simulink model "passive_cell_balancing"  (R2017b)
settings: Solver=VariableStepAuto  StartTime=0.0  StopTime=500  MaxStep=1e-4  RelTol=1e-3
undefined symbols (not defined in the file): Hydride, Metal, Nickel
libraries: powerlib x7, electricdrivelib x3
settings Model: Creator=DELL  LastModifiedBy=DELL

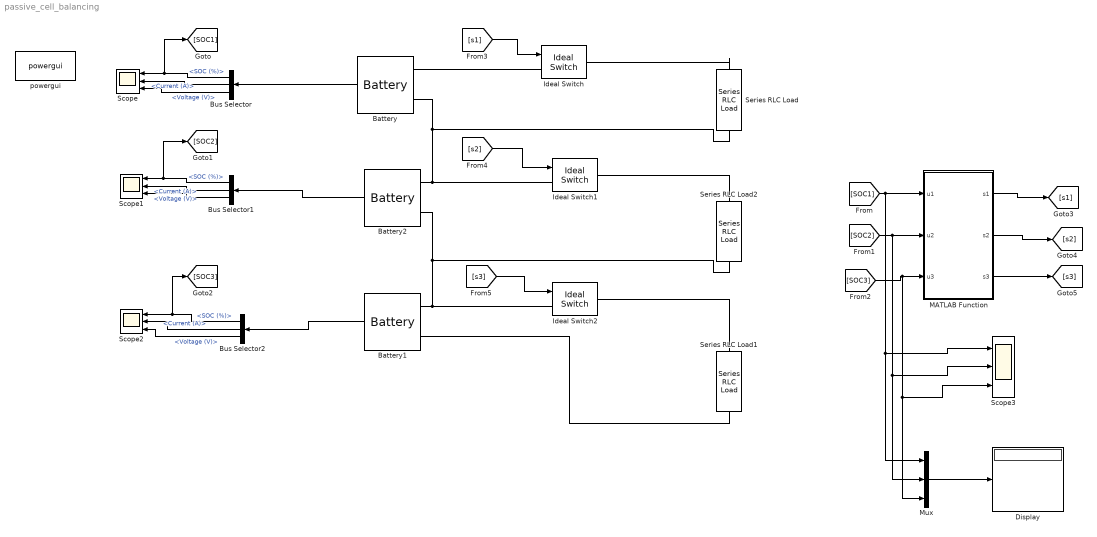
== system passive_cell_balancing ==
  Battery : electricdrivelib/Extra Sources/Battery  BatType=Nickel-Metal-Hydride  ShowTempParam=off  ThermalPreset=no  ShowAgeParam=off  NomV=7.2  NomQ=6.5  SOC=60  Batt_Tr=1  PresetModel=off  MaxQ=5.4  MinV=5.4  FullV=8.3807  Dis_rate=2.3478  R=0.013333  Normal_OP=4.8835  expZone="[7.7788      0.2653]"  current=[6.5 13 32.5]  Units=Time  Tci=20  NomT=20  T2=-30  MaxQ2=4.8  FullV2=7.1  Normal_OP2=5.655  expZone2="[6.58           1]"  Rca=0.6  ti=2000  Dp=0  Neq0=0  Tsim=1e6  Ta1=25  Qeol=5.4*0.9  Reol=0.013333*1.2  Char_age=[2.3478, 3]  Dis_age=[2.3478, 10]  N1=1500  N2=10500  N3=1000  N4=1400  Ta2=45  N5=950
  Battery1 : electricdrivelib/Extra Sources/Battery  BatType=Nickel-Metal-Hydride  ShowTempParam=off  ThermalPreset=no  ShowAgeParam=off  NomV=7.2  NomQ=6.5  SOC=55  Batt_Tr=1  PresetModel=off  MaxQ=5.4  MinV=5.4  FullV=8.3807  Dis_rate=2.3478  R=0.013333  Normal_OP=4.8835  expZone="[7.7788      0.2653]"  current=[6.5 13 32.5]  Units=Time  Tci=20  NomT=20  T2=-30  MaxQ2=4.8  FullV2=7.1  Normal_OP2=5.655  expZone2="[6.58           1]"  Rca=0.6  ti=2000  Dp=0  Neq0=0  Tsim=1e6  Ta1=25  Qeol=5.4*0.9  Reol=0.013333*1.2  Char_age=[2.3478, 3]  Dis_age=[2.3478, 10]  N1=1500  N2=10500  N3=1000  N4=1400  Ta2=45  N5=950
  Battery2 : electricdrivelib/Extra Sources/Battery  BatType=Nickel-Metal-Hydride  ShowTempParam=off  ThermalPreset=no  ShowAgeParam=off  NomV=7.2  NomQ=6.5  SOC=50  Batt_Tr=1  PresetModel=off  MaxQ=5.4  MinV=5.4  FullV=8.3807  Dis_rate=2.3478  R=0.013333  Normal_OP=4.8835  expZone="[7.7788      0.2653]"  current=[6.5 13 32.5]  Units=Time  Tci=20  NomT=20  T2=-30  MaxQ2=4.8  FullV2=7.1  Normal_OP2=5.655  expZone2="[6.58           1]"  Rca=0.6  ti=2000  Dp=0  Neq0=0  Tsim=1e6  Ta1=25  Qeol=5.4*0.9  Reol=0.013333*1.2  Char_age=[2.3478, 3]  Dis_age=[2.3478, 10]  N1=1500  N2=10500  N3=1000  N4=1400  Ta2=45  N5=950
  Bus Selector : BusSelector  OutputSignals=SOC (%),Current (A),Voltage (V)
  Bus Selector1 : BusSelector  OutputSignals=SOC (%),Current (A),Voltage (V)
  Bus Selector2 : BusSelector  OutputSignals=SOC (%),Current (A),Voltage (V)
  Display : Display
  Ideal Switch : powerlib/Power Electronics/Ideal Switch  Ron=0.001  Lon=0  IC=0  Rs=1e5  Cs=inf  Measurements=off
  Ideal Switch1 : powerlib/Power Electronics/Ideal Switch  Ron=0.001  Lon=0  IC=0  Rs=1e5  Cs=inf  Measurements=off
  Ideal Switch2 : powerlib/Power Electronics/Ideal Switch  Ron=0.001  Lon=0  IC=0  Rs=1e5  Cs=inf  Measurements=off
  MATLAB Function : MATLAB Function  TreatAsAtomicUnit=on
  Mux : Mux  Inputs=3
  Scope{,1..3} (4 alike) : Scope  NumInputPorts=3
  Series RLC Load : powerlib/Elements/Series RLC Load  LConnTagsString=a  RConnTagsString=__new0  NominalVoltage=8  NominalFrequency=0.1  ActivePower=1000  InductivePower=0  CapacitivePower=0  Setx0=off  InitialVoltage=0  SetiL0=off  InitialCurrent=0  Measurements=None  LoadType=constant Z
  Series RLC Load1 : powerlib/Elements/Series RLC Load  LConnTagsString=a  RConnTagsString=__new0  NominalVoltage=8  NominalFrequency=0.1  ActivePower=1000  InductivePower=0  CapacitivePower=0  Setx0=off  InitialVoltage=0  SetiL0=off  InitialCurrent=0  Measurements=None  LoadType=constant Z
  Series RLC Load2 : powerlib/Elements/Series RLC Load  LConnTagsString=a  RConnTagsString=__new0  NominalVoltage=8  NominalFrequency=0.1  ActivePower=1000  InductivePower=0  CapacitivePower=0  Setx0=off  InitialVoltage=0  SetiL0=off  InitialCurrent=0  Measurements=None  LoadType=constant Z
  powergui : powerlib/powergui  Priority=1  SimulationMode=Continuous  SampleTime=50e-6  frequency=60  Iterations=50  frequencyindice=0  Pbase=100e6  ErrMax=1e-4  UnitsV=kV  UnitsW=MW  buscounter=0  FunctionMessages=off  echomessages=off  EnableUseOfTLC=off  CurrentSourceSwitches=off  DisableSnubberDevices=off  DisableRonSwitches=off  DisableVfSwitches=off  DisplayEquations=off  SolverType=Tustin/Backward Euler (TBE)  Interpol=off  ExternalGateDelay=off  methode=off  Ts=100  x0status=blocks  SPID=on  SwTol=0  HookPort=off  RestoreLinks=warning  ResistiveCurrentMeasurement=off  Frange=[0:2:500]  Ylog=off  Xlog=on  ShowGrid=off  save=off  variable=ZData  structure=0  ZoomFFT=off  StartTime=0.0  cycles=1  DisplayStyle=1  fundamental=60  FreqAxis=off  MaxFrequency=1000  frequencyindicesteady=1  RmsSteady=1  display=off
  wires:
  Battery/1 -> Bus Selector/1
  Battery2/1 -> Bus Selector1/1
  Battery1/1 -> Bus Selector2/1
  Bus Selector/1 -> [SOC1], Scope/1  "<SOC (%)>"
  Bus Selector/2 -> Scope/2  "<Current (A)>"
  Bus Selector/3 -> Scope/3  "<Voltage (V)>"
  Bus Selector1/1 -> [SOC2], Scope1/1  "<SOC (%)>"
  Bus Selector1/2 -> Scope1/2  "<Current (A)>"
  Bus Selector1/3 -> Scope1/3  "<Voltage (V)>"
  Bus Selector2/1 -> [SOC3], Scope2/1  "<SOC (%)>"
  Bus Selector2/2 -> Scope2/2  "<Current (A)>"
  Bus Selector2/3 -> Scope2/3  "<Voltage (V)>"
  [SOC2] -> Scope3/2, Mux/2, MATLAB Function/2(u2)
  [SOC3] -> Scope3/3, Mux/3, MATLAB Function/3(u3)
  MATLAB Function/1(s1) -> [s1]
  MATLAB Function/2(s2) -> [s2]
  MATLAB Function/3(s3) -> [s3]
  [s1] -> Ideal Switch/1
  [s2] -> Ideal Switch1/1
  [s3] -> Ideal Switch2/1
  [SOC1] -> Scope3/1, Mux/1, MATLAB Function/1(u1)
  Mux/1 -> Display/1
  connections:
  Battery/LConn2 -- Series RLC Load/RConn1 -- Ideal Switch1/LConn1 -- Battery2/LConn1
  Battery2/LConn2 -- Series RLC Load2/RConn1 -- Ideal Switch2/LConn1 -- Battery1/LConn1
  Ideal Switch/LConn1 -- Battery/LConn1
  Series RLC Load/LConn1 -- Ideal Switch/RConn1
  Series RLC Load2/LConn1 -- Ideal Switch1/RConn1
  Series RLC Load1/LConn1 -- Ideal Switch2/RConn1
  Series RLC Load1/RConn1 -- Battery1/LConn2

== matlab function passive_cell_balancing/MATLAB Function ==
  data: u1 input; s1 output; u2 input; u3 input; s2 output; s3 output
function [s1,s2,s3] = fcn(u1,u2,u3)

u1=int32(u1)
u2=int32(u2)
u3=int32(u3)

if((u1>u2) || (u1>u3))
     s1=1;
else
     s1=0;
end

if((u2>u1) || (u2>u3))
     s2=1;
else
     s2=0;
end
    
if((u3>u1) || (u3>u2))
     s3=1;
else
     s3=0;
end
